simulink model "task4"  (R2023b)
settings: Solver=VariableStepAuto  StartTime=0.0  StopTime=10.0  RelTol=1e-3

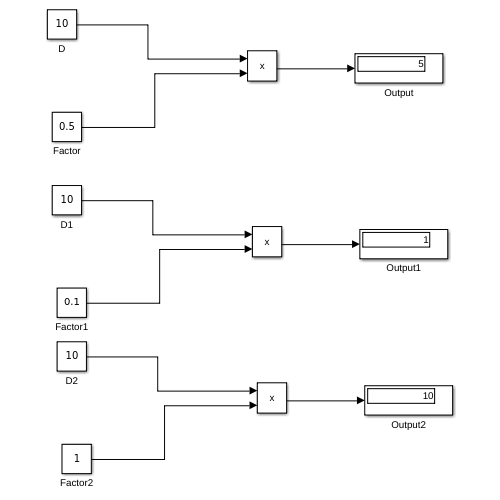
[thumbnail: Simulink's stored preview of the top-level diagram]
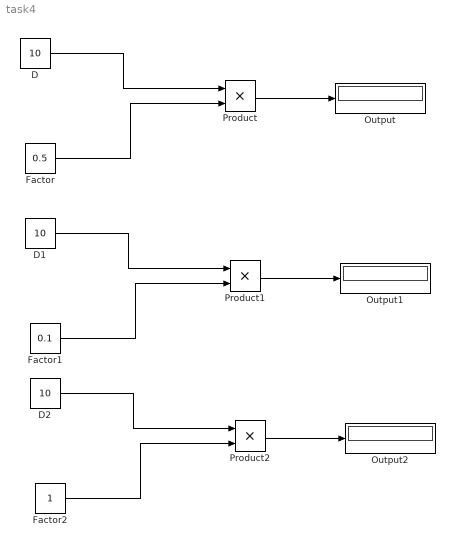
== system task4 ==
  D : Constant  Value=10
  D1 : Constant  Value=10
  D2 : Constant  Value=10
  Factor : Constant  Value=0.5
  Factor1 : Constant  Value=0.1
  Factor2 : Constant
  Output : Display
  Output1 : Display
  Output2 : Display
  Product : Product
  Product1 : Product
  Product2 : Product
  wires:
  D/1 -> Product/1
  Product/1 -> Output/1
  Factor/1 -> Product/2
  D1/1 -> Product1/1
  Factor1/1 -> Product1/2
  Product1/1 -> Output1/1
  D2/1 -> Product2/1
  Factor2/1 -> Product2/2
  Product2/1 -> Output2/1
